simulink model "Controllers"  (R2015a)
settings: Solver=ode45  SolverMode=SingleTasking  StartTime=0.0  StopTime=10.0  RelTol=1e-3
undefined symbols (not defined in the file): mA, mB, mC, mD, mK, mL
libraries: simulink x2
settings Model: CovMetricSettings=dwe  CovHtmlReporting=off  covSaveCumulativeToWorkspaceVar=off  CovSaveSingleToWorkspaceVar=off  CovExternalEMLEnable=on  Creator=insha  LastModifiedBy=insha
settings DataIOCC: LimitDataPoints=off  SaveFormat=Dataset  ReturnWorkspaceOutputs=on
settings DebuggingCC: SFUnexpectedBacktrackingDiag=error  SFNoUnconditionalDefaultTransitionDiag=error
settings HardwareCC: ProdBitPerPointer=64  ProdLargestAtomicFloat=Float  ProdIntDivRoundTo=Zero  ProdEndianess=LittleEndian  ProdHWDeviceType=Specified
settings ModelReferenceCC: PropagateSignalLabelsOutOfModel=on
settings SFSimCC: SimUseLocalCustomCode=on
settings RTWCC: RTWUseLocalCustomCode=on
settings GRTTargetCC: TargetLangStandard=C99 (ISO)

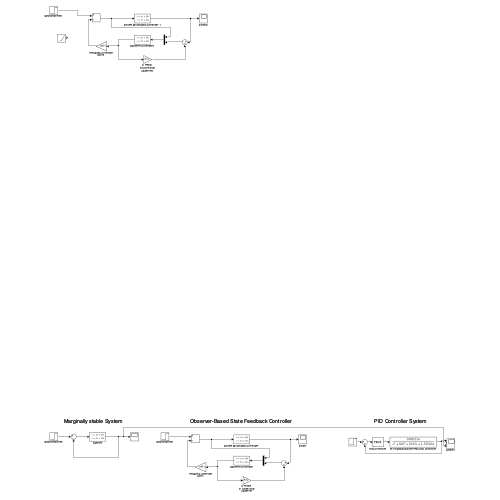
[thumbnail: Simulink's stored preview of the top-level diagram]
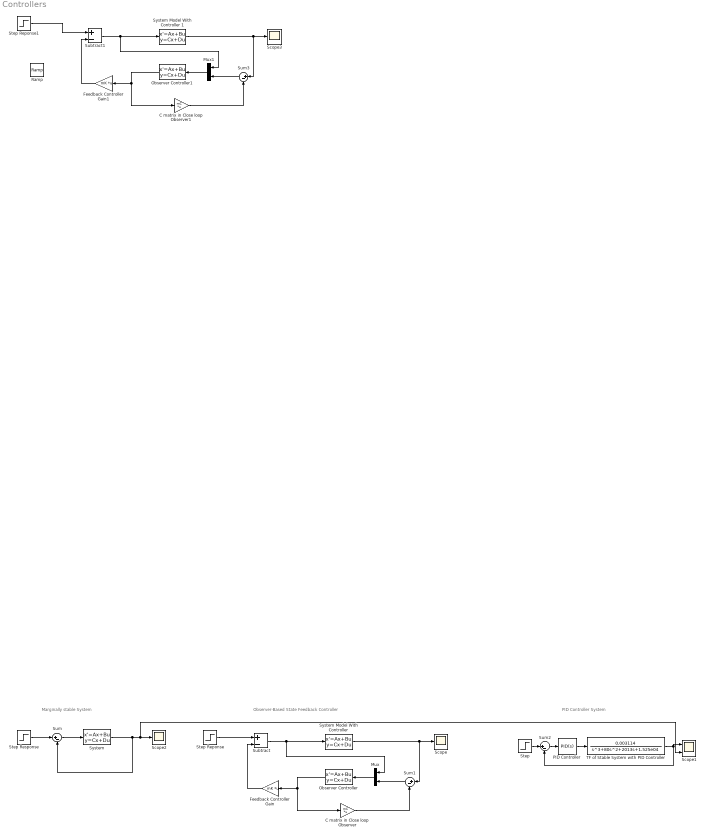
== system Controllers ==
  note: PID Controller System
  note: Marginally stable System
  note: Observer-Based State Feedback Controller
  " System" : StateSpace  A=mA  B=mB  C=mC  D=mD  X0=0
  C matrix in Close loop Observer : Gain  Gain=mC  Multiplication=Matrix(K*u)
  C matrix in Close loop Observer1 : Gain  Gain=mC  Multiplication=Matrix(K*u)
  Feedback Controller Gain : Gain  Gain=mK  Multiplication=Matrix(K*u)
  Feedback Controller Gain1 : Gain  Gain=mK  Multiplication=Matrix(K*u)
  Mux : Mux  Inputs=2
  Mux1 : Mux  Inputs=2
  Observer Controller : StateSpace  A=mA  B=[mB mL]  C=[1 0 0; 0 1 0; 0 0 1]  D=[0 0;0 0;0 0]  X0=0
  Observer Controller1 : StateSpace  A=mA  B=[mB mL]  C=[1 0 0; 0 1 0; 0 0 1]  D=[0 0;0 0;0 0]  X0=0
  PID Controller : simulink/Continuous/PID Controller  Controller=PID  Form=Parallel  TimeDomain=Continuous-time  SampleTime=-1  IntegratorMethod=Forward Euler  FilterMethod=Forward Euler  ControllerParametersSource=internal  P=10599414.9219599  I=83189948.7980299  D=335136.517629795  UseFilter=on  N=2140.45218900231  InitialConditionSource=internal  InitialConditionForIntegrator=0  InitialConditionForFilter=0  DifferentiatorICPrevScaledInput=0  ExternalReset=none  TrackingMode=off  Kt=1  LimitOutput=off  UpperSaturationLimit=inf  LowerSaturationLimit=-inf  LinearizeAsGain=on  AntiWindupMode=none  Kb=1  POutMin=[]  POutMax=[]  IOutMin=[]  IOutMax=[]  DOutMin=[]  DOutMax=[]  NOutMin=[]  NOutMax=[]  SumOutMin=[]  SumOutMax=[]  SaturationOutMin=[]  SaturationOutMax=[]  PParamMin=[]  PParamMax=[]  IParamMin=[]  IParamMax=[]  DParamMin=[]  DParamMax=[]  NParamMin=[]  NParamMax=[]  KbParamMin=[]  KbParamMax=[]  KtParamMin=[]  KtParamMax=[]  KbOutMin=[]  KbOutMax=[]  KtOutMin=[]  KtOutMax=[]  IntegratorOutMin=[]  IntegratorOutMax=[]  FilterOutMin=[]  FilterOutMax=[]  SumI1OutMin=[]  SumI1OutMax=[]  SumI2OutMin=[]  SumI2OutMax=[]  SumI3OutMin=[]  SumI3OutMax=[]  SumDOutMin=[]  SumDOutMax=[]  DifferentiatorOutMin=[]  DifferentiatorOutMax=[]  IntegratorContinuousStateAttributes=''  IntegratorStateMustResolveToSignalObject=off  IntegratorRTWStateStorageClass=Auto  FilterContinuousStateAttributes=''  FilterStateMustResolveToSignalObject=off  FilterRTWStateStorageClass=Auto
  Ramp : simulink/Sources/Ramp  slope=5  start=0  X0=0
  Scope : Scope
      settings: TimeRange=auto  ShowLegends=on  MaxDataPoints=5000  SaveToWorkspace=off  SaveName=ScopeData  YMin=-0.00000003  YMax=0.00000023  SampleTime=-1
  Scope1 : Scope  NumInputPorts=3
      settings: TimeRange=auto  TickLabels=on  ShowLegends=on  MaxDataPoints=5000  SaveToWorkspace=off  SaveName=ScopeData2  YMin=-0.125~-5~-5  YMax=1.125~5~5  SampleTime=-1
  Scope2 : Scope
      settings: TimeRange=auto  ShowLegends=on  MaxDataPoints=5000  SaveToWorkspace=off  YMin=-0.0018  YMax=0.0162  SampleTime=-1
  Scope3 : Scope
      settings: TimeRange=auto  ShowLegends=on  MaxDataPoints=5000  SaveToWorkspace=off  YMin=-0.0000001  YMax=0.0000011  SampleTime=-1
  Step : Step  SampleTime=0
  Step Reponse : Step  SampleTime=0
  Step Reponse1 : Step  After=5  SampleTime=0
  Step Response : Step  SampleTime=0
  Subtract : Sum  Inputs=+-
  Subtract1 : Sum  Inputs=+-
  Sum{,1..3} (4 alike) : Sum  Inputs=|+-
  "System Model With Controller " : StateSpace  A=mA  B=mB  C=mC  D=mD  X0=0
  System Model With Controller 1 : StateSpace  A=mA  B=mB  C=mC  D=mD  X0=0
  TF of Stable System with PID Controller : TransferFcn  Numerator=[0.003114]  Denominator=[1 80 2013 1.525e04]
  wires:
  "System Model With Controller "/1 -> Sum1/1, Scope/1
  Step Reponse/1 -> Subtract/1
  Subtract/1 -> Mux/1, "System Model With Controller "/1
  C matrix in Close loop Observer/1 -> Sum1/2
  Mux/1 -> Observer Controller/1
  Observer Controller/1 -> C matrix in Close loop Observer/1, Feedback Controller Gain/1
  Feedback Controller Gain/1 -> Subtract/2
  Sum1/1 -> Mux/2
  Step Response/1 -> Sum/1
  Sum/1 -> " System"/1
  " System"/1 -> Scope1/3, Scope2/1, Sum/2
  TF of Stable System with PID Controller/1 -> Sum2/2, Scope1/1
  Step/1 -> Sum2/1
  Sum2/1 -> PID Controller/1
  PID Controller/1 -> TF of Stable System with PID Controller/1
  Feedback Controller Gain1/1 -> Subtract1/2
  Subtract1/1 -> Mux1/1, System Model With Controller 1/1
  C matrix in Close loop Observer1/1 -> Sum3/2
  System Model With Controller 1/1 -> Sum3/1, Scope3/1
  Observer Controller1/1 -> C matrix in Close loop Observer1/1, Feedback Controller Gain1/1
  Sum3/1 -> Mux1/2
  Mux1/1 -> Observer Controller1/1
  Step Reponse1/1 -> Subtract1/1
